simulink model "GunnerusDP_v1"  (R2017b)
settings: Solver=ode4  StartTime=0.0  StopTime=Tsim  FixedStep=ts  RelTol=1e-3  EnableMultiTasking=on
values from neighbouring files (symbols this model uses):
  ts = 0.01    [InitGunnerusDP.m]
undefined symbols (not defined in the file or in its folder): Control, Current, Hoerner, Par, Sim, TC_currentChange, vessel, vesselABC
libraries: marine_hydro x4, marine_gnc x3, simulink x3
(part 3 of 4)

== system GunnerusDP_v1/Environment and Vessel Dynamics/Wave definiton (from MCSim)/wave height and wave frequency/Hs and omega20/hs ==
  time : Inport
  Constant : Constant  Value=v1
  Constant2 : Constant  Value=v2
  If : If  IfExpression=u1 < t1  ElseIfExpressions=u1>=t1 & u1<t2
  If Action Subsystem1 : Subsystem  TreatAsAtomicUnit=on
  If Action Subsystem2 : Subsystem  TreatAsAtomicUnit=on
  If Action Subsystem3 : Subsystem  TreatAsAtomicUnit=on
  Merge : Merge  Inputs=3
  omega_peak : Outport
  wires:
  time/1 -> If Action Subsystem2/1(In1), If/1
  If/3 -> If Action Subsystem3/Action
  If/1 -> If Action Subsystem1/Action
  Constant/1 -> If Action Subsystem1/1(In1)
  Constant2/1 -> If Action Subsystem3/1(In1)
  If Action Subsystem3/1(Out1) -> Merge/3
  If Action Subsystem2/1(Out1) -> Merge/2
  If/2 -> If Action Subsystem2/Action
  If Action Subsystem1/1(Out1) -> Merge/1
  Merge/1 -> omega_peak/1

== system GunnerusDP_v1/Environment and Vessel Dynamics/Wave definiton (from MCSim)/wave height and wave frequency/Hs and omega20/omega_p ==
  time : Inport
  Constant : Constant  Value=v1
  Constant2 : Constant  Value=v2
  If : If  IfExpression=u1 < t1  ElseIfExpressions=u1>=t1 & u1<t2
  If Action Subsystem1 : Subsystem  TreatAsAtomicUnit=on
  If Action Subsystem2 : Subsystem  TreatAsAtomicUnit=on
  If Action Subsystem3 : Subsystem  TreatAsAtomicUnit=on
  Merge : Merge  Inputs=3
  omega_peak : Outport
  wires:
  Merge/1 -> omega_peak/1
  If Action Subsystem1/1(Out1) -> Merge/1
  If/2 -> If Action Subsystem2/Action
  If Action Subsystem2/1(Out1) -> Merge/2
  If Action Subsystem3/1(Out1) -> Merge/3
  Constant2/1 -> If Action Subsystem3/1(In1)
  Constant/1 -> If Action Subsystem1/1(In1)
  If/1 -> If Action Subsystem1/Action
  If/3 -> If Action Subsystem3/Action
  time/1 -> If/1, If Action Subsystem2/1(In1)

== system GunnerusDP_v1/Environment and Vessel Dynamics/Wave definiton (from MCSim)/wave height and wave frequency/Hs and omega21/hs ==
  time : Inport
  Constant : Constant  Value=v1
  Constant2 : Constant  Value=v2
  If : If  IfExpression=u1 < t1  ElseIfExpressions=u1>=t1 & u1<t2
  If Action Subsystem1 : Subsystem  TreatAsAtomicUnit=on
  If Action Subsystem2 : Subsystem  TreatAsAtomicUnit=on
  If Action Subsystem3 : Subsystem  TreatAsAtomicUnit=on
  Merge : Merge  Inputs=3
  omega_peak : Outport
  wires:
  Merge/1 -> omega_peak/1
  If Action Subsystem1/1(Out1) -> Merge/1
  If/2 -> If Action Subsystem2/Action
  If Action Subsystem2/1(Out1) -> Merge/2
  If Action Subsystem3/1(Out1) -> Merge/3
  Constant2/1 -> If Action Subsystem3/1(In1)
  Constant/1 -> If Action Subsystem1/1(In1)
  If/1 -> If Action Subsystem1/Action
  If/3 -> If Action Subsystem3/Action
  time/1 -> If/1, If Action Subsystem2/1(In1)

== system GunnerusDP_v1/Environment and Vessel Dynamics/Wave definiton (from MCSim)/wave height and wave frequency/Hs and omega21/omega_p ==
  time : Inport
  Constant : Constant  Value=v1
  Constant2 : Constant  Value=v2
  If : If  IfExpression=u1 < t1  ElseIfExpressions=u1>=t1 & u1<t2
  If Action Subsystem1 : Subsystem  TreatAsAtomicUnit=on
  If Action Subsystem2 : Subsystem  TreatAsAtomicUnit=on
  If Action Subsystem3 : Subsystem  TreatAsAtomicUnit=on
  Merge : Merge  Inputs=3
  omega_peak : Outport
  wires:
  time/1 -> If Action Subsystem2/1(In1), If/1
  If/3 -> If Action Subsystem3/Action
  If/1 -> If Action Subsystem1/Action
  Constant/1 -> If Action Subsystem1/1(In1)
  Constant2/1 -> If Action Subsystem3/1(In1)
  If Action Subsystem3/1(Out1) -> Merge/3
  If Action Subsystem2/1(Out1) -> Merge/2
  If/2 -> If Action Subsystem2/Action
  If Action Subsystem1/1(Out1) -> Merge/1
  Merge/1 -> omega_peak/1

== system GunnerusDP_v1/Environment and Vessel Dynamics/Wave definiton (from MCSim)/wave height and wave frequency/Hs and omega22/hs ==
  time : Inport
  Constant : Constant  Value=v1
  Constant2 : Constant  Value=v2
  If : If  IfExpression=u1 < t1  ElseIfExpressions=u1>=t1 & u1<t2
  If Action Subsystem1 : Subsystem  TreatAsAtomicUnit=on
  If Action Subsystem2 : Subsystem  TreatAsAtomicUnit=on
  If Action Subsystem3 : Subsystem  TreatAsAtomicUnit=on
  Merge : Merge  Inputs=3
  omega_peak : Outport
  wires:
  time/1 -> If Action Subsystem2/1(In1), If/1
  If/3 -> If Action Subsystem3/Action
  If/1 -> If Action Subsystem1/Action
  Constant/1 -> If Action Subsystem1/1(In1)
  Constant2/1 -> If Action Subsystem3/1(In1)
  If Action Subsystem3/1(Out1) -> Merge/3
  If Action Subsystem2/1(Out1) -> Merge/2
  If/2 -> If Action Subsystem2/Action
  If Action Subsystem1/1(Out1) -> Merge/1
  Merge/1 -> omega_peak/1

== system GunnerusDP_v1/Environment and Vessel Dynamics/Wave definiton (from MCSim)/wave height and wave frequency/Hs and omega22/omega_p ==
  time : Inport
  Constant : Constant  Value=v1
  Constant2 : Constant  Value=v2
  If : If  IfExpression=u1 < t1  ElseIfExpressions=u1>=t1 & u1<t2
  If Action Subsystem1 : Subsystem  TreatAsAtomicUnit=on
  If Action Subsystem2 : Subsystem  TreatAsAtomicUnit=on
  If Action Subsystem3 : Subsystem  TreatAsAtomicUnit=on
  Merge : Merge  Inputs=3
  omega_peak : Outport
  wires:
  Merge/1 -> omega_peak/1
  If Action Subsystem1/1(Out1) -> Merge/1
  If/2 -> If Action Subsystem2/Action
  If Action Subsystem2/1(Out1) -> Merge/2
  If Action Subsystem3/1(Out1) -> Merge/3
  Constant2/1 -> If Action Subsystem3/1(In1)
  Constant/1 -> If Action Subsystem1/1(In1)
  If/1 -> If Action Subsystem1/Action
  If/3 -> If Action Subsystem3/Action
  time/1 -> If/1, If Action Subsystem2/1(In1)

== system GunnerusDP_v1/Environment and Vessel Dynamics/Wave definiton (from MCSim)/wave height and wave frequency/Hs and omega23/hs ==
  time : Inport
  Constant : Constant  Value=v1
  Constant2 : Constant  Value=v2
  If : If  IfExpression=u1 < t1  ElseIfExpressions=u1>=t1 & u1<t2
  If Action Subsystem1 : Subsystem  TreatAsAtomicUnit=on
  If Action Subsystem2 : Subsystem  TreatAsAtomicUnit=on
  If Action Subsystem3 : Subsystem  TreatAsAtomicUnit=on
  Merge : Merge  Inputs=3
  omega_peak : Outport
  wires:
  Merge/1 -> omega_peak/1
  If Action Subsystem1/1(Out1) -> Merge/1
  If/2 -> If Action Subsystem2/Action
  If Action Subsystem2/1(Out1) -> Merge/2
  If Action Subsystem3/1(Out1) -> Merge/3
  Constant2/1 -> If Action Subsystem3/1(In1)
  Constant/1 -> If Action Subsystem1/1(In1)
  If/1 -> If Action Subsystem1/Action
  If/3 -> If Action Subsystem3/Action
  time/1 -> If/1, If Action Subsystem2/1(In1)

== system GunnerusDP_v1/Environment and Vessel Dynamics/Wave definiton (from MCSim)/wave height and wave frequency/Hs and omega23/omega_p ==
  time : Inport
  Constant : Constant  Value=v1
  Constant2 : Constant  Value=v2
  If : If  IfExpression=u1 < t1  ElseIfExpressions=u1>=t1 & u1<t2
  If Action Subsystem1 : Subsystem  TreatAsAtomicUnit=on
  If Action Subsystem2 : Subsystem  TreatAsAtomicUnit=on
  If Action Subsystem3 : Subsystem  TreatAsAtomicUnit=on
  Merge : Merge  Inputs=3
  omega_peak : Outport
  wires:
  time/1 -> If Action Subsystem2/1(In1), If/1
  If/3 -> If Action Subsystem3/Action
  If/1 -> If Action Subsystem1/Action
  Constant/1 -> If Action Subsystem1/1(In1)
  Constant2/1 -> If Action Subsystem3/1(In1)
  If Action Subsystem3/1(Out1) -> Merge/3
  If Action Subsystem2/1(Out1) -> Merge/2
  If/2 -> If Action Subsystem2/Action
  If Action Subsystem1/1(Out1) -> Merge/1
  Merge/1 -> omega_peak/1

== system GunnerusDP_v1/Environment and Vessel Dynamics/Wave definiton (from MCSim)/wave height and wave frequency/Hs and omega24/hs ==
  time : Inport
  Constant : Constant  Value=v1
  Constant2 : Constant  Value=v2
  If : If  IfExpression=u1 < t1  ElseIfExpressions=u1>=t1 & u1<t2
  If Action Subsystem1 : Subsystem  TreatAsAtomicUnit=on
  If Action Subsystem2 : Subsystem  TreatAsAtomicUnit=on
  If Action Subsystem3 : Subsystem  TreatAsAtomicUnit=on
  Merge : Merge  Inputs=3
  omega_peak : Outport
  wires:
  time/1 -> If Action Subsystem2/1(In1), If/1
  If/3 -> If Action Subsystem3/Action
  If/1 -> If Action Subsystem1/Action
  Constant/1 -> If Action Subsystem1/1(In1)
  Constant2/1 -> If Action Subsystem3/1(In1)
  If Action Subsystem3/1(Out1) -> Merge/3
  If Action Subsystem2/1(Out1) -> Merge/2
  If/2 -> If Action Subsystem2/Action
  If Action Subsystem1/1(Out1) -> Merge/1
  Merge/1 -> omega_peak/1

== system GunnerusDP_v1/Environment and Vessel Dynamics/Wave definiton (from MCSim)/wave height and wave frequency/Hs and omega24/omega_p ==
  time : Inport
  Constant : Constant  Value=v1
  Constant2 : Constant  Value=v2
  If : If  IfExpression=u1 < t1  ElseIfExpressions=u1>=t1 & u1<t2
  If Action Subsystem1 : Subsystem  TreatAsAtomicUnit=on
  If Action Subsystem2 : Subsystem  TreatAsAtomicUnit=on
  If Action Subsystem3 : Subsystem  TreatAsAtomicUnit=on
  Merge : Merge  Inputs=3
  omega_peak : Outport
  wires:
  Merge/1 -> omega_peak/1
  If Action Subsystem1/1(Out1) -> Merge/1
  If/2 -> If Action Subsystem2/Action
  If Action Subsystem2/1(Out1) -> Merge/2
  If Action Subsystem3/1(Out1) -> Merge/3
  Constant2/1 -> If Action Subsystem3/1(In1)
  Constant/1 -> If Action Subsystem1/1(In1)
  If/1 -> If Action Subsystem1/Action
  If/3 -> If Action Subsystem3/Action
  time/1 -> If/1, If Action Subsystem2/1(In1)

== system GunnerusDP_v1/Environment and Vessel Dynamics/Wave definiton (from MCSim)/wave height and wave frequency/Hs and omega3/hs ==
  time : Inport
  Constant : Constant  Value=v1
  Constant2 : Constant  Value=v2
  If : If  IfExpression=u1 < t1  ElseIfExpressions=u1>=t1 & u1<t2
  If Action Subsystem1 : Subsystem  TreatAsAtomicUnit=on
  If Action Subsystem2 : Subsystem  TreatAsAtomicUnit=on
  If Action Subsystem3 : Subsystem  TreatAsAtomicUnit=on
  Merge : Merge  Inputs=3
  omega_peak : Outport
  wires:
  time/1 -> If Action Subsystem2/1(In1), If/1
  If/3 -> If Action Subsystem3/Action
  If/1 -> If Action Subsystem1/Action
  Constant/1 -> If Action Subsystem1/1(In1)
  Constant2/1 -> If Action Subsystem3/1(In1)
  If Action Subsystem3/1(Out1) -> Merge/3
  If Action Subsystem2/1(Out1) -> Merge/2
  If/2 -> If Action Subsystem2/Action
  If Action Subsystem1/1(Out1) -> Merge/1
  Merge/1 -> omega_peak/1

== system GunnerusDP_v1/Environment and Vessel Dynamics/Wave definiton (from MCSim)/wave height and wave frequency/Hs and omega3/omega_p ==
  time : Inport
  Constant : Constant  Value=v1
  Constant2 : Constant  Value=v2
  If : If  IfExpression=u1 < t1  ElseIfExpressions=u1>=t1 & u1<t2
  If Action Subsystem1 : Subsystem  TreatAsAtomicUnit=on
  If Action Subsystem2 : Subsystem  TreatAsAtomicUnit=on
  If Action Subsystem3 : Subsystem  TreatAsAtomicUnit=on
  Merge : Merge  Inputs=3
  omega_peak : Outport
  wires:
  Merge/1 -> omega_peak/1
  If Action Subsystem1/1(Out1) -> Merge/1
  If/2 -> If Action Subsystem2/Action
  If Action Subsystem2/1(Out1) -> Merge/2
  If Action Subsystem3/1(Out1) -> Merge/3
  Constant2/1 -> If Action Subsystem3/1(In1)
  Constant/1 -> If Action Subsystem1/1(In1)
  If/1 -> If Action Subsystem1/Action
  If/3 -> If Action Subsystem3/Action
  time/1 -> If/1, If Action Subsystem2/1(In1)

== system GunnerusDP_v1/Environment and Vessel Dynamics/Wave definiton (from MCSim)/wave height and wave frequency/Hs and omega4/hs ==
  time : Inport
  Constant : Constant  Value=v1
  Constant2 : Constant  Value=v2
  If : If  IfExpression=u1 < t1  ElseIfExpressions=u1>=t1 & u1<t2
  If Action Subsystem1 : Subsystem  TreatAsAtomicUnit=on
  If Action Subsystem2 : Subsystem  TreatAsAtomicUnit=on
  If Action Subsystem3 : Subsystem  TreatAsAtomicUnit=on
  Merge : Merge  Inputs=3
  omega_peak : Outport
  wires:
  Merge/1 -> omega_peak/1
  If Action Subsystem1/1(Out1) -> Merge/1
  If/2 -> If Action Subsystem2/Action
  If Action Subsystem2/1(Out1) -> Merge/2
  If Action Subsystem3/1(Out1) -> Merge/3
  Constant2/1 -> If Action Subsystem3/1(In1)
  Constant/1 -> If Action Subsystem1/1(In1)
  If/1 -> If Action Subsystem1/Action
  If/3 -> If Action Subsystem3/Action
  time/1 -> If/1, If Action Subsystem2/1(In1)

== system GunnerusDP_v1/Environment and Vessel Dynamics/Wave definiton (from MCSim)/wave height and wave frequency/Hs and omega4/omega_p ==
  time : Inport
  Constant : Constant  Value=v1
  Constant2 : Constant  Value=v2
  If : If  IfExpression=u1 < t1  ElseIfExpressions=u1>=t1 & u1<t2
  If Action Subsystem1 : Subsystem  TreatAsAtomicUnit=on
  If Action Subsystem2 : Subsystem  TreatAsAtomicUnit=on
  If Action Subsystem3 : Subsystem  TreatAsAtomicUnit=on
  Merge : Merge  Inputs=3
  omega_peak : Outport
  wires:
  time/1 -> If Action Subsystem2/1(In1), If/1
  If/3 -> If Action Subsystem3/Action
  If/1 -> If Action Subsystem1/Action
  Constant/1 -> If Action Subsystem1/1(In1)
  Constant2/1 -> If Action Subsystem3/1(In1)
  If Action Subsystem3/1(Out1) -> Merge/3
  If Action Subsystem2/1(Out1) -> Merge/2
  If/2 -> If Action Subsystem2/Action
  If Action Subsystem1/1(Out1) -> Merge/1
  Merge/1 -> omega_peak/1

== system GunnerusDP_v1/Environment and Vessel Dynamics/Wave definiton (from MCSim)/wave height and wave frequency/Hs and omega5/hs ==
  time : Inport
  Constant : Constant  Value=v1
  Constant2 : Constant  Value=v2
  If : If  IfExpression=u1 < t1  ElseIfExpressions=u1>=t1 & u1<t2
  If Action Subsystem1 : Subsystem  TreatAsAtomicUnit=on
  If Action Subsystem2 : Subsystem  TreatAsAtomicUnit=on
  If Action Subsystem3 : Subsystem  TreatAsAtomicUnit=on
  Merge : Merge  Inputs=3
  omega_peak : Outport
  wires:
  time/1 -> If Action Subsystem2/1(In1), If/1
  If/3 -> If Action Subsystem3/Action
  If/1 -> If Action Subsystem1/Action
  Constant/1 -> If Action Subsystem1/1(In1)
  Constant2/1 -> If Action Subsystem3/1(In1)
  If Action Subsystem3/1(Out1) -> Merge/3
  If Action Subsystem2/1(Out1) -> Merge/2
  If/2 -> If Action Subsystem2/Action
  If Action Subsystem1/1(Out1) -> Merge/1
  Merge/1 -> omega_peak/1

== system GunnerusDP_v1/Environment and Vessel Dynamics/Wave definiton (from MCSim)/wave height and wave frequency/Hs and omega5/omega_p ==
  time : Inport
  Constant : Constant  Value=v1
  Constant2 : Constant  Value=v2
  If : If  IfExpression=u1 < t1  ElseIfExpressions=u1>=t1 & u1<t2
  If Action Subsystem1 : Subsystem  TreatAsAtomicUnit=on
  If Action Subsystem2 : Subsystem  TreatAsAtomicUnit=on
  If Action Subsystem3 : Subsystem  TreatAsAtomicUnit=on
  Merge : Merge  Inputs=3
  omega_peak : Outport
  wires:
  Merge/1 -> omega_peak/1
  If Action Subsystem1/1(Out1) -> Merge/1
  If/2 -> If Action Subsystem2/Action
  If Action Subsystem2/1(Out1) -> Merge/2
  If Action Subsystem3/1(Out1) -> Merge/3
  Constant2/1 -> If Action Subsystem3/1(In1)
  Constant/1 -> If Action Subsystem1/1(In1)
  If/1 -> If Action Subsystem1/Action
  If/3 -> If Action Subsystem3/Action
  time/1 -> If/1, If Action Subsystem2/1(In1)

== system GunnerusDP_v1/Environment and Vessel Dynamics/Wave definiton (from MCSim)/wave height and wave frequency/Hs and omega6/hs ==
  time : Inport
  Constant : Constant  Value=v1
  Constant2 : Constant  Value=v2
  If : If  IfExpression=u1 < t1  ElseIfExpressions=u1>=t1 & u1<t2
  If Action Subsystem1 : Subsystem  TreatAsAtomicUnit=on
  If Action Subsystem2 : Subsystem  TreatAsAtomicUnit=on
  If Action Subsystem3 : Subsystem  TreatAsAtomicUnit=on
  Merge : Merge  Inputs=3
  omega_peak : Outport
  wires:
  Merge/1 -> omega_peak/1
  If Action Subsystem1/1(Out1) -> Merge/1
  If/2 -> If Action Subsystem2/Action
  If Action Subsystem2/1(Out1) -> Merge/2
  If Action Subsystem3/1(Out1) -> Merge/3
  Constant2/1 -> If Action Subsystem3/1(In1)
  Constant/1 -> If Action Subsystem1/1(In1)
  If/1 -> If Action Subsystem1/Action
  If/3 -> If Action Subsystem3/Action
  time/1 -> If/1, If Action Subsystem2/1(In1)

== system GunnerusDP_v1/Environment and Vessel Dynamics/Wave definiton (from MCSim)/wave height and wave frequency/Hs and omega6/omega_p ==
  time : Inport
  Constant : Constant  Value=v1
  Constant2 : Constant  Value=v2
  If : If  IfExpression=u1 < t1  ElseIfExpressions=u1>=t1 & u1<t2
  If Action Subsystem1 : Subsystem  TreatAsAtomicUnit=on
  If Action Subsystem2 : Subsystem  TreatAsAtomicUnit=on
  If Action Subsystem3 : Subsystem  TreatAsAtomicUnit=on
  Merge : Merge  Inputs=3
  omega_peak : Outport
  wires:
  time/1 -> If Action Subsystem2/1(In1), If/1
  If/3 -> If Action Subsystem3/Action
  If/1 -> If Action Subsystem1/Action
  Constant/1 -> If Action Subsystem1/1(In1)
  Constant2/1 -> If Action Subsystem3/1(In1)
  If Action Subsystem3/1(Out1) -> Merge/3
  If Action Subsystem2/1(Out1) -> Merge/2
  If/2 -> If Action Subsystem2/Action
  If Action Subsystem1/1(Out1) -> Merge/1
  Merge/1 -> omega_peak/1

== system GunnerusDP_v1/Environment and Vessel Dynamics/Wave definiton (from MCSim)/wave height and wave frequency/Hs and omega7/hs ==
  time : Inport
  Constant : Constant  Value=v1
  Constant2 : Constant  Value=v2
  If : If  IfExpression=u1 < t1  ElseIfExpressions=u1>=t1 & u1<t2
  If Action Subsystem1 : Subsystem  TreatAsAtomicUnit=on
  If Action Subsystem2 : Subsystem  TreatAsAtomicUnit=on
  If Action Subsystem3 : Subsystem  TreatAsAtomicUnit=on
  Merge : Merge  Inputs=3
  omega_peak : Outport
  wires:
  time/1 -> If Action Subsystem2/1(In1), If/1
  If/3 -> If Action Subsystem3/Action
  If/1 -> If Action Subsystem1/Action
  Constant/1 -> If Action Subsystem1/1(In1)
  Constant2/1 -> If Action Subsystem3/1(In1)
  If Action Subsystem3/1(Out1) -> Merge/3
  If Action Subsystem2/1(Out1) -> Merge/2
  If/2 -> If Action Subsystem2/Action
  If Action Subsystem1/1(Out1) -> Merge/1
  Merge/1 -> omega_peak/1

== system GunnerusDP_v1/Environment and Vessel Dynamics/Wave definiton (from MCSim)/wave height and wave frequency/Hs and omega7/omega_p ==
  time : Inport
  Constant : Constant  Value=v1
  Constant2 : Constant  Value=v2
  If : If  IfExpression=u1 < t1  ElseIfExpressions=u1>=t1 & u1<t2
  If Action Subsystem1 : Subsystem  TreatAsAtomicUnit=on
  If Action Subsystem2 : Subsystem  TreatAsAtomicUnit=on
  If Action Subsystem3 : Subsystem  TreatAsAtomicUnit=on
  Merge : Merge  Inputs=3
  omega_peak : Outport
  wires:
  Merge/1 -> omega_peak/1
  If Action Subsystem1/1(Out1) -> Merge/1
  If/2 -> If Action Subsystem2/Action
  If Action Subsystem2/1(Out1) -> Merge/2
  If Action Subsystem3/1(Out1) -> Merge/3
  Constant2/1 -> If Action Subsystem3/1(In1)
  Constant/1 -> If Action Subsystem1/1(In1)
  If/1 -> If Action Subsystem1/Action
  If/3 -> If Action Subsystem3/Action
  time/1 -> If/1, If Action Subsystem2/1(In1)

== system GunnerusDP_v1/Environment and Vessel Dynamics/Wave definiton (from MCSim)/wave height and wave frequency/Hs and omega8/hs ==
  time : Inport
  Constant : Constant  Value=v1
  Constant2 : Constant  Value=v2
  If : If  IfExpression=u1 < t1  ElseIfExpressions=u1>=t1 & u1<t2
  If Action Subsystem1 : Subsystem  TreatAsAtomicUnit=on
  If Action Subsystem2 : Subsystem  TreatAsAtomicUnit=on
  If Action Subsystem3 : Subsystem  TreatAsAtomicUnit=on
  Merge : Merge  Inputs=3
  omega_peak : Outport
  wires:
  Merge/1 -> omega_peak/1
  If Action Subsystem1/1(Out1) -> Merge/1
  If/2 -> If Action Subsystem2/Action
  If Action Subsystem2/1(Out1) -> Merge/2
  If Action Subsystem3/1(Out1) -> Merge/3
  Constant2/1 -> If Action Subsystem3/1(In1)
  Constant/1 -> If Action Subsystem1/1(In1)
  If/1 -> If Action Subsystem1/Action
  If/3 -> If Action Subsystem3/Action
  time/1 -> If/1, If Action Subsystem2/1(In1)

== system GunnerusDP_v1/Environment and Vessel Dynamics/Wave definiton (from MCSim)/wave height and wave frequency/Hs and omega8/omega_p ==
  time : Inport
  Constant : Constant  Value=v1
  Constant2 : Constant  Value=v2
  If : If  IfExpression=u1 < t1  ElseIfExpressions=u1>=t1 & u1<t2
  If Action Subsystem1 : Subsystem  TreatAsAtomicUnit=on
  If Action Subsystem2 : Subsystem  TreatAsAtomicUnit=on
  If Action Subsystem3 : Subsystem  TreatAsAtomicUnit=on
  Merge : Merge  Inputs=3
  omega_peak : Outport
  wires:
  time/1 -> If Action Subsystem2/1(In1), If/1
  If/3 -> If Action Subsystem3/Action
  If/1 -> If Action Subsystem1/Action
  Constant/1 -> If Action Subsystem1/1(In1)
  Constant2/1 -> If Action Subsystem3/1(In1)
  If Action Subsystem3/1(Out1) -> Merge/3
  If Action Subsystem2/1(Out1) -> Merge/2
  If/2 -> If Action Subsystem2/Action
  If Action Subsystem1/1(Out1) -> Merge/1
  Merge/1 -> omega_peak/1

== system GunnerusDP_v1/Environment and Vessel Dynamics/Wave definiton (from MCSim)/wave height and wave frequency/Hs and omega9/hs ==
  time : Inport
  Constant : Constant  Value=v1
  Constant2 : Constant  Value=v2
  If : If  IfExpression=u1 < t1  ElseIfExpressions=u1>=t1 & u1<t2
  If Action Subsystem1 : Subsystem  TreatAsAtomicUnit=on
  If Action Subsystem2 : Subsystem  TreatAsAtomicUnit=on
  If Action Subsystem3 : Subsystem  TreatAsAtomicUnit=on
  Merge : Merge  Inputs=3
  omega_peak : Outport
  wires:
  time/1 -> If Action Subsystem2/1(In1), If/1
  If/3 -> If Action Subsystem3/Action
  If/1 -> If Action Subsystem1/Action
  Constant/1 -> If Action Subsystem1/1(In1)
  Constant2/1 -> If Action Subsystem3/1(In1)
  If Action Subsystem3/1(Out1) -> Merge/3
  If Action Subsystem2/1(Out1) -> Merge/2
  If/2 -> If Action Subsystem2/Action
  If Action Subsystem1/1(Out1) -> Merge/1
  Merge/1 -> omega_peak/1

== system GunnerusDP_v1/Environment and Vessel Dynamics/Wave definiton (from MCSim)/wave height and wave frequency/Hs and omega9/omega_p ==
  time : Inport
  Constant : Constant  Value=v1
  Constant2 : Constant  Value=v2
  If : If  IfExpression=u1 < t1  ElseIfExpressions=u1>=t1 & u1<t2
  If Action Subsystem1 : Subsystem  TreatAsAtomicUnit=on
  If Action Subsystem2 : Subsystem  TreatAsAtomicUnit=on
  If Action Subsystem3 : Subsystem  TreatAsAtomicUnit=on
  Merge : Merge  Inputs=3
  omega_peak : Outport
  wires:
  Merge/1 -> omega_peak/1
  If Action Subsystem1/1(Out1) -> Merge/1
  If/2 -> If Action Subsystem2/Action
  If Action Subsystem2/1(Out1) -> Merge/2
  If Action Subsystem3/1(Out1) -> Merge/3
  Constant2/1 -> If Action Subsystem3/1(In1)
  Constant/1 -> If Action Subsystem1/1(In1)
  If/1 -> If Action Subsystem1/Action
  If/3 -> If Action Subsystem3/Action
  time/1 -> If/1, If Action Subsystem2/1(In1)

== system GunnerusDP_v1/Environment and Vessel Dynamics/Wave definiton (from MCSim)/wave height and wave frequency/Hs and omega1/hs/If Action Subsystem1 ==
  In1 : Inport
  Action Port : ActionPort  ActionType=then
  Out1 : Outport
  wires:
  In1/1 -> Out1/1

== system GunnerusDP_v1/Environment and Vessel Dynamics/Wave definiton (from MCSim)/wave height and wave frequency/Hs and omega1/hs/If Action Subsystem2 ==
  In1 : Inport
  Action Port : ActionPort  ActionType=elseif
  Fcn : Fcn  Expr=v1-(v1-v2)/(t2-t1)*(u[1]-t1)
  Out1 : Outport
  wires:
  In1/1 -> Fcn/1
  Fcn/1 -> Out1/1

== system GunnerusDP_v1/Environment and Vessel Dynamics/Wave definiton (from MCSim)/wave height and wave frequency/Hs and omega1/hs/If Action Subsystem3 ==
  In1 : Inport
  Action Port : ActionPort  ActionType=else
  Out1 : Outport
  wires:
  In1/1 -> Out1/1

== system GunnerusDP_v1/Environment and Vessel Dynamics/Wave definiton (from MCSim)/wave height and wave frequency/Hs and omega1/omega_p/If Action Subsystem1 ==
  In1 : Inport
  Action Port : ActionPort  ActionType=then
  Out1 : Outport
  wires:
  In1/1 -> Out1/1

== system GunnerusDP_v1/Environment and Vessel Dynamics/Wave definiton (from MCSim)/wave height and wave frequency/Hs and omega1/omega_p/If Action Subsystem2 ==
  In1 : Inport
  Action Port : ActionPort  ActionType=elseif
  Fcn : Fcn  Expr=v1-(v1-v2)/(t2-t1)*(u[1]-t1)
  Out1 : Outport
  wires:
  Fcn/1 -> Out1/1
  In1/1 -> Fcn/1

== system GunnerusDP_v1/Environment and Vessel Dynamics/Wave definiton (from MCSim)/wave height and wave frequency/Hs and omega1/omega_p/If Action Subsystem3 ==
  In1 : Inport
  Action Port : ActionPort  ActionType=else
  Out1 : Outport
  wires:
  In1/1 -> Out1/1

== system GunnerusDP_v1/Environment and Vessel Dynamics/Wave definiton (from MCSim)/wave height and wave frequency/Hs and omega10/hs/If Action Subsystem1 ==
  In1 : Inport
  Action Port : ActionPort  ActionType=then
  Out1 : Outport
  wires:
  In1/1 -> Out1/1

== system GunnerusDP_v1/Environment and Vessel Dynamics/Wave definiton (from MCSim)/wave height and wave frequency/Hs and omega10/hs/If Action Subsystem2 ==
  In1 : Inport
  Action Port : ActionPort  ActionType=elseif
  Fcn : Fcn  Expr=v1-(v1-v2)/(t2-t1)*(u[1]-t1)
  Out1 : Outport
  wires:
  Fcn/1 -> Out1/1
  In1/1 -> Fcn/1

== system GunnerusDP_v1/Environment and Vessel Dynamics/Wave definiton (from MCSim)/wave height and wave frequency/Hs and omega10/hs/If Action Subsystem3 ==
  In1 : Inport
  Action Port : ActionPort  ActionType=else
  Out1 : Outport
  wires:
  In1/1 -> Out1/1

== system GunnerusDP_v1/Environment and Vessel Dynamics/Wave definiton (from MCSim)/wave height and wave frequency/Hs and omega10/omega_p/If Action Subsystem1 ==
  In1 : Inport
  Action Port : ActionPort  ActionType=then
  Out1 : Outport
  wires:
  In1/1 -> Out1/1

== system GunnerusDP_v1/Environment and Vessel Dynamics/Wave definiton (from MCSim)/wave height and wave frequency/Hs and omega10/omega_p/If Action Subsystem2 ==
  In1 : Inport
  Action Port : ActionPort  ActionType=elseif
  Fcn : Fcn  Expr=v1-(v1-v2)/(t2-t1)*(u[1]-t1)
  Out1 : Outport
  wires:
  In1/1 -> Fcn/1
  Fcn/1 -> Out1/1

== system GunnerusDP_v1/Environment and Vessel Dynamics/Wave definiton (from MCSim)/wave height and wave frequency/Hs and omega10/omega_p/If Action Subsystem3 ==
  In1 : Inport
  Action Port : ActionPort  ActionType=else
  Out1 : Outport
  wires:
  In1/1 -> Out1/1

== system GunnerusDP_v1/Environment and Vessel Dynamics/Wave definiton (from MCSim)/wave height and wave frequency/Hs and omega11/hs/If Action Subsystem1 ==
  In1 : Inport
  Action Port : ActionPort  ActionType=then
  Out1 : Outport
  wires:
  In1/1 -> Out1/1

== system GunnerusDP_v1/Environment and Vessel Dynamics/Wave definiton (from MCSim)/wave height and wave frequency/Hs and omega11/hs/If Action Subsystem2 ==
  In1 : Inport
  Action Port : ActionPort  ActionType=elseif
  Fcn : Fcn  Expr=v1-(v1-v2)/(t2-t1)*(u[1]-t1)
  Out1 : Outport
  wires:
  In1/1 -> Fcn/1
  Fcn/1 -> Out1/1

== system GunnerusDP_v1/Environment and Vessel Dynamics/Wave definiton (from MCSim)/wave height and wave frequency/Hs and omega11/hs/If Action Subsystem3 ==
  In1 : Inport
  Action Port : ActionPort  ActionType=else
  Out1 : Outport
  wires:
  In1/1 -> Out1/1

== system GunnerusDP_v1/Environment and Vessel Dynamics/Wave definiton (from MCSim)/wave height and wave frequency/Hs and omega11/omega_p/If Action Subsystem1 ==
  In1 : Inport
  Action Port : ActionPort  ActionType=then
  Out1 : Outport
  wires:
  In1/1 -> Out1/1

== system GunnerusDP_v1/Environment and Vessel Dynamics/Wave definiton (from MCSim)/wave height and wave frequency/Hs and omega11/omega_p/If Action Subsystem2 ==
  In1 : Inport
  Action Port : ActionPort  ActionType=elseif
  Fcn : Fcn  Expr=v1-(v1-v2)/(t2-t1)*(u[1]-t1)
  Out1 : Outport
  wires:
  Fcn/1 -> Out1/1
  In1/1 -> Fcn/1

== system GunnerusDP_v1/Environment and Vessel Dynamics/Wave definiton (from MCSim)/wave height and wave frequency/Hs and omega11/omega_p/If Action Subsystem3 ==
  In1 : Inport
  Action Port : ActionPort  ActionType=else
  Out1 : Outport
  wires:
  In1/1 -> Out1/1

== system GunnerusDP_v1/Environment and Vessel Dynamics/Wave definiton (from MCSim)/wave height and wave frequency/Hs and omega12/hs/If Action Subsystem1 ==
  In1 : Inport
  Action Port : ActionPort  ActionType=then
  Out1 : Outport
  wires:
  In1/1 -> Out1/1

== system GunnerusDP_v1/Environment and Vessel Dynamics/Wave definiton (from MCSim)/wave height and wave frequency/Hs and omega12/hs/If Action Subsystem2 ==
  In1 : Inport
  Action Port : ActionPort  ActionType=elseif
  Fcn : Fcn  Expr=v1-(v1-v2)/(t2-t1)*(u[1]-t1)
  Out1 : Outport
  wires:
  Fcn/1 -> Out1/1
  In1/1 -> Fcn/1

== system GunnerusDP_v1/Environment and Vessel Dynamics/Wave definiton (from MCSim)/wave height and wave frequency/Hs and omega12/hs/If Action Subsystem3 ==
  In1 : Inport
  Action Port : ActionPort  ActionType=else
  Out1 : Outport
  wires:
  In1/1 -> Out1/1

== system GunnerusDP_v1/Environment and Vessel Dynamics/Wave definiton (from MCSim)/wave height and wave frequency/Hs and omega12/omega_p/If Action Subsystem1 ==
  In1 : Inport
  Action Port : ActionPort  ActionType=then
  Out1 : Outport
  wires:
  In1/1 -> Out1/1

== system GunnerusDP_v1/Environment and Vessel Dynamics/Wave definiton (from MCSim)/wave height and wave frequency/Hs and omega12/omega_p/If Action Subsystem2 ==
  In1 : Inport
  Action Port : ActionPort  ActionType=elseif
  Fcn : Fcn  Expr=v1-(v1-v2)/(t2-t1)*(u[1]-t1)
  Out1 : Outport
  wires:
  In1/1 -> Fcn/1
  Fcn/1 -> Out1/1

== system GunnerusDP_v1/Environment and Vessel Dynamics/Wave definiton (from MCSim)/wave height and wave frequency/Hs and omega12/omega_p/If Action Subsystem3 ==
  In1 : Inport
  Action Port : ActionPort  ActionType=else
  Out1 : Outport
  wires:
  In1/1 -> Out1/1

== system GunnerusDP_v1/Environment and Vessel Dynamics/Wave definiton (from MCSim)/wave height and wave frequency/Hs and omega13/hs/If Action Subsystem1 ==
  In1 : Inport
  Action Port : ActionPort  ActionType=then
  Out1 : Outport
  wires:
  In1/1 -> Out1/1

== system GunnerusDP_v1/Environment and Vessel Dynamics/Wave definiton (from MCSim)/wave height and wave frequency/Hs and omega13/hs/If Action Subsystem2 ==
  In1 : Inport
  Action Port : ActionPort  ActionType=elseif
  Fcn : Fcn  Expr=v1-(v1-v2)/(t2-t1)*(u[1]-t1)
  Out1 : Outport
  wires:
  In1/1 -> Fcn/1
  Fcn/1 -> Out1/1

== system GunnerusDP_v1/Environment and Vessel Dynamics/Wave definiton (from MCSim)/wave height and wave frequency/Hs and omega13/hs/If Action Subsystem3 ==
  In1 : Inport
  Action Port : ActionPort  ActionType=else
  Out1 : Outport
  wires:
  In1/1 -> Out1/1

== system GunnerusDP_v1/Environment and Vessel Dynamics/Wave definiton (from MCSim)/wave height and wave frequency/Hs and omega13/omega_p/If Action Subsystem1 ==
  In1 : Inport
  Action Port : ActionPort  ActionType=then
  Out1 : Outport
  wires:
  In1/1 -> Out1/1

== system GunnerusDP_v1/Environment and Vessel Dynamics/Wave definiton (from MCSim)/wave height and wave frequency/Hs and omega13/omega_p/If Action Subsystem2 ==
  In1 : Inport
  Action Port : ActionPort  ActionType=elseif
  Fcn : Fcn  Expr=v1-(v1-v2)/(t2-t1)*(u[1]-t1)
  Out1 : Outport
  wires:
  Fcn/1 -> Out1/1
  In1/1 -> Fcn/1

== system GunnerusDP_v1/Environment and Vessel Dynamics/Wave definiton (from MCSim)/wave height and wave frequency/Hs and omega13/omega_p/If Action Subsystem3 ==
  In1 : Inport
  Action Port : ActionPort  ActionType=else
  Out1 : Outport
  wires:
  In1/1 -> Out1/1

== system GunnerusDP_v1/Environment and Vessel Dynamics/Wave definiton (from MCSim)/wave height and wave frequency/Hs and omega14/hs/If Action Subsystem1 ==
  In1 : Inport
  Action Port : ActionPort  ActionType=then
  Out1 : Outport
  wires:
  In1/1 -> Out1/1

== system GunnerusDP_v1/Environment and Vessel Dynamics/Wave definiton (from MCSim)/wave height and wave frequency/Hs and omega14/hs/If Action Subsystem2 ==
  In1 : Inport
  Action Port : ActionPort  ActionType=elseif
  Fcn : Fcn  Expr=v1-(v1-v2)/(t2-t1)*(u[1]-t1)
  Out1 : Outport
  wires:
  Fcn/1 -> Out1/1
  In1/1 -> Fcn/1

== system GunnerusDP_v1/Environment and Vessel Dynamics/Wave definiton (from MCSim)/wave height and wave frequency/Hs and omega14/hs/If Action Subsystem3 ==
  In1 : Inport
  Action Port : ActionPort  ActionType=else
  Out1 : Outport
  wires:
  In1/1 -> Out1/1

== system GunnerusDP_v1/Environment and Vessel Dynamics/Wave definiton (from MCSim)/wave height and wave frequency/Hs and omega14/omega_p/If Action Subsystem1 ==
  In1 : Inport
  Action Port : ActionPort  ActionType=then
  Out1 : Outport
  wires:
  In1/1 -> Out1/1

== system GunnerusDP_v1/Environment and Vessel Dynamics/Wave definiton (from MCSim)/wave height and wave frequency/Hs and omega14/omega_p/If Action Subsystem2 ==
  In1 : Inport
  Action Port : ActionPort  ActionType=elseif
  Fcn : Fcn  Expr=v1-(v1-v2)/(t2-t1)*(u[1]-t1)
  Out1 : Outport
  wires:
  In1/1 -> Fcn/1
  Fcn/1 -> Out1/1

== system GunnerusDP_v1/Environment and Vessel Dynamics/Wave definiton (from MCSim)/wave height and wave frequency/Hs and omega14/omega_p/If Action Subsystem3 ==
  In1 : Inport
  Action Port : ActionPort  ActionType=else
  Out1 : Outport
  wires:
  In1/1 -> Out1/1

== system GunnerusDP_v1/Environment and Vessel Dynamics/Wave definiton (from MCSim)/wave height and wave frequency/Hs and omega15/hs/If Action Subsystem1 ==
  In1 : Inport
  Action Port : ActionPort  ActionType=then
  Out1 : Outport
  wires:
  In1/1 -> Out1/1

== system GunnerusDP_v1/Environment and Vessel Dynamics/Wave definiton (from MCSim)/wave height and wave frequency/Hs and omega15/hs/If Action Subsystem2 ==
  In1 : Inport
  Action Port : ActionPort  ActionType=elseif
  Fcn : Fcn  Expr=v1-(v1-v2)/(t2-t1)*(u[1]-t1)
  Out1 : Outport
  wires:
  In1/1 -> Fcn/1
  Fcn/1 -> Out1/1

== system GunnerusDP_v1/Environment and Vessel Dynamics/Wave definiton (from MCSim)/wave height and wave frequency/Hs and omega15/hs/If Action Subsystem3 ==
  In1 : Inport
  Action Port : ActionPort  ActionType=else
  Out1 : Outport
  wires:
  In1/1 -> Out1/1

== system GunnerusDP_v1/Environment and Vessel Dynamics/Wave definiton (from MCSim)/wave height and wave frequency/Hs and omega15/omega_p/If Action Subsystem1 ==
  In1 : Inport
  Action Port : ActionPort  ActionType=then
  Out1 : Outport
  wires:
  In1/1 -> Out1/1

== system GunnerusDP_v1/Environment and Vessel Dynamics/Wave definiton (from MCSim)/wave height and wave frequency/Hs and omega15/omega_p/If Action Subsystem2 ==
  In1 : Inport
  Action Port : ActionPort  ActionType=elseif
  Fcn : Fcn  Expr=v1-(v1-v2)/(t2-t1)*(u[1]-t1)
  Out1 : Outport
  wires:
  Fcn/1 -> Out1/1
  In1/1 -> Fcn/1

== system GunnerusDP_v1/Environment and Vessel Dynamics/Wave definiton (from MCSim)/wave height and wave frequency/Hs and omega15/omega_p/If Action Subsystem3 ==
  In1 : Inport
  Action Port : ActionPort  ActionType=else
  Out1 : Outport
  wires:
  In1/1 -> Out1/1

== system GunnerusDP_v1/Environment and Vessel Dynamics/Wave definiton (from MCSim)/wave height and wave frequency/Hs and omega16/hs/If Action Subsystem1 ==
  In1 : Inport
  Action Port : ActionPort  ActionType=then
  Out1 : Outport
  wires:
  In1/1 -> Out1/1

== system GunnerusDP_v1/Environment and Vessel Dynamics/Wave definiton (from MCSim)/wave height and wave frequency/Hs and omega16/hs/If Action Subsystem2 ==
  In1 : Inport
  Action Port : ActionPort  ActionType=elseif
  Fcn : Fcn  Expr=v1-(v1-v2)/(t2-t1)*(u[1]-t1)
  Out1 : Outport
  wires:
  In1/1 -> Fcn/1
  Fcn/1 -> Out1/1

== system GunnerusDP_v1/Environment and Vessel Dynamics/Wave definiton (from MCSim)/wave height and wave frequency/Hs and omega16/hs/If Action Subsystem3 ==
  In1 : Inport
  Action Port : ActionPort  ActionType=else
  Out1 : Outport
  wires:
  In1/1 -> Out1/1

== system GunnerusDP_v1/Environment and Vessel Dynamics/Wave definiton (from MCSim)/wave height and wave frequency/Hs and omega16/omega_p/If Action Subsystem1 ==
  In1 : Inport
  Action Port : ActionPort  ActionType=then
  Out1 : Outport
  wires:
  In1/1 -> Out1/1

== system GunnerusDP_v1/Environment and Vessel Dynamics/Wave definiton (from MCSim)/wave height and wave frequency/Hs and omega16/omega_p/If Action Subsystem2 ==
  In1 : Inport
  Action Port : ActionPort  ActionType=elseif
  Fcn : Fcn  Expr=v1-(v1-v2)/(t2-t1)*(u[1]-t1)
  Out1 : Outport
  wires:
  Fcn/1 -> Out1/1
  In1/1 -> Fcn/1

== system GunnerusDP_v1/Environment and Vessel Dynamics/Wave definiton (from MCSim)/wave height and wave frequency/Hs and omega16/omega_p/If Action Subsystem3 ==
  In1 : Inport
  Action Port : ActionPort  ActionType=else
  Out1 : Outport
  wires:
  In1/1 -> Out1/1

== system GunnerusDP_v1/Environment and Vessel Dynamics/Wave definiton (from MCSim)/wave height and wave frequency/Hs and omega17/hs/If Action Subsystem1 ==
  In1 : Inport
  Action Port : ActionPort  ActionType=then
  Out1 : Outport
  wires:
  In1/1 -> Out1/1

== system GunnerusDP_v1/Environment and Vessel Dynamics/Wave definiton (from MCSim)/wave height and wave frequency/Hs and omega17/hs/If Action Subsystem2 ==
  In1 : Inport
  Action Port : ActionPort  ActionType=elseif
  Fcn : Fcn  Expr=v1-(v1-v2)/(t2-t1)*(u[1]-t1)
  Out1 : Outport
  wires:
  Fcn/1 -> Out1/1
  In1/1 -> Fcn/1

== system GunnerusDP_v1/Environment and Vessel Dynamics/Wave definiton (from MCSim)/wave height and wave frequency/Hs and omega17/hs/If Action Subsystem3 ==
  In1 : Inport
  Action Port : ActionPort  ActionType=else
  Out1 : Outport
  wires:
  In1/1 -> Out1/1

== system GunnerusDP_v1/Environment and Vessel Dynamics/Wave definiton (from MCSim)/wave height and wave frequency/Hs and omega17/omega_p/If Action Subsystem1 ==
  In1 : Inport
  Action Port : ActionPort  ActionType=then
  Out1 : Outport
  wires:
  In1/1 -> Out1/1

== system GunnerusDP_v1/Environment and Vessel Dynamics/Wave definiton (from MCSim)/wave height and wave frequency/Hs and omega17/omega_p/If Action Subsystem2 ==
  In1 : Inport
  Action Port : ActionPort  ActionType=elseif
  Fcn : Fcn  Expr=v1-(v1-v2)/(t2-t1)*(u[1]-t1)
  Out1 : Outport
  wires:
  In1/1 -> Fcn/1
  Fcn/1 -> Out1/1

== system GunnerusDP_v1/Environment and Vessel Dynamics/Wave definiton (from MCSim)/wave height and wave frequency/Hs and omega17/omega_p/If Action Subsystem3 ==
  In1 : Inport
  Action Port : ActionPort  ActionType=else
  Out1 : Outport
  wires:
  In1/1 -> Out1/1

== system GunnerusDP_v1/Environment and Vessel Dynamics/Wave definiton (from MCSim)/wave height and wave frequency/Hs and omega18/hs/If Action Subsystem1 ==
  In1 : Inport
  Action Port : ActionPort  ActionType=then
  Out1 : Outport
  wires:
  In1/1 -> Out1/1

== system GunnerusDP_v1/Environment and Vessel Dynamics/Wave definiton (from MCSim)/wave height and wave frequency/Hs and omega18/hs/If Action Subsystem2 ==
  In1 : Inport
  Action Port : ActionPort  ActionType=elseif
  Fcn : Fcn  Expr=v1-(v1-v2)/(t2-t1)*(u[1]-t1)
  Out1 : Outport
  wires:
  In1/1 -> Fcn/1
  Fcn/1 -> Out1/1

== system GunnerusDP_v1/Environment and Vessel Dynamics/Wave definiton (from MCSim)/wave height and wave frequency/Hs and omega18/hs/If Action Subsystem3 ==
  In1 : Inport
  Action Port : ActionPort  ActionType=else
  Out1 : Outport
  wires:
  In1/1 -> Out1/1

== system GunnerusDP_v1/Environment and Vessel Dynamics/Wave definiton (from MCSim)/wave height and wave frequency/Hs and omega18/omega_p/If Action Subsystem1 ==
  In1 : Inport
  Action Port : ActionPort  ActionType=then
  Out1 : Outport
  wires:
  In1/1 -> Out1/1

== system GunnerusDP_v1/Environment and Vessel Dynamics/Wave definiton (from MCSim)/wave height and wave frequency/Hs and omega18/omega_p/If Action Subsystem2 ==
  In1 : Inport
  Action Port : ActionPort  ActionType=elseif
  Fcn : Fcn  Expr=v1-(v1-v2)/(t2-t1)*(u[1]-t1)
  Out1 : Outport
  wires:
  Fcn/1 -> Out1/1
  In1/1 -> Fcn/1

== system GunnerusDP_v1/Environment and Vessel Dynamics/Wave definiton (from MCSim)/wave height and wave frequency/Hs and omega18/omega_p/If Action Subsystem3 ==
  In1 : Inport
  Action Port : ActionPort  ActionType=else
  Out1 : Outport
  wires:
  In1/1 -> Out1/1

== system GunnerusDP_v1/Environment and Vessel Dynamics/Wave definiton (from MCSim)/wave height and wave frequency/Hs and omega19/hs/If Action Subsystem1 ==
  In1 : Inport
  Action Port : ActionPort  ActionType=then
  Out1 : Outport
  wires:
  In1/1 -> Out1/1

== system GunnerusDP_v1/Environment and Vessel Dynamics/Wave definiton (from MCSim)/wave height and wave frequency/Hs and omega19/hs/If Action Subsystem2 ==
  In1 : Inport
  Action Port : ActionPort  ActionType=elseif
  Fcn : Fcn  Expr=v1-(v1-v2)/(t2-t1)*(u[1]-t1)
  Out1 : Outport
  wires:
  Fcn/1 -> Out1/1
  In1/1 -> Fcn/1

== system GunnerusDP_v1/Environment and Vessel Dynamics/Wave definiton (from MCSim)/wave height and wave frequency/Hs and omega19/hs/If Action Subsystem3 ==
  In1 : Inport
  Action Port : ActionPort  ActionType=else
  Out1 : Outport
  wires:
  In1/1 -> Out1/1

== system GunnerusDP_v1/Environment and Vessel Dynamics/Wave definiton (from MCSim)/wave height and wave frequency/Hs and omega19/omega_p/If Action Subsystem1 ==
  In1 : Inport
  Action Port : ActionPort  ActionType=then
  Out1 : Outport
  wires:
  In1/1 -> Out1/1

== system GunnerusDP_v1/Environment and Vessel Dynamics/Wave definiton (from MCSim)/wave height and wave frequency/Hs and omega19/omega_p/If Action Subsystem2 ==
  In1 : Inport
  Action Port : ActionPort  ActionType=elseif
  Fcn : Fcn  Expr=v1-(v1-v2)/(t2-t1)*(u[1]-t1)
  Out1 : Outport
  wires:
  In1/1 -> Fcn/1
  Fcn/1 -> Out1/1

== system GunnerusDP_v1/Environment and Vessel Dynamics/Wave definiton (from MCSim)/wave height and wave frequency/Hs and omega19/omega_p/If Action Subsystem3 ==
  In1 : Inport
  Action Port : ActionPort  ActionType=else
  Out1 : Outport
  wires:
  In1/1 -> Out1/1

== system GunnerusDP_v1/Environment and Vessel Dynamics/Wave definiton (from MCSim)/wave height and wave frequency/Hs and omega2/hs/If Action Subsystem1 ==
  In1 : Inport
  Action Port : ActionPort  ActionType=then
  Out1 : Outport
  wires:
  In1/1 -> Out1/1

== system GunnerusDP_v1/Environment and Vessel Dynamics/Wave definiton (from MCSim)/wave height and wave frequency/Hs and omega2/hs/If Action Subsystem2 ==
  In1 : Inport
  Action Port : ActionPort  ActionType=elseif
  Fcn : Fcn  Expr=v1-(v1-v2)/(t2-t1)*(u[1]-t1)
  Out1 : Outport
  wires:
  Fcn/1 -> Out1/1
  In1/1 -> Fcn/1

== system GunnerusDP_v1/Environment and Vessel Dynamics/Wave definiton (from MCSim)/wave height and wave frequency/Hs and omega2/hs/If Action Subsystem3 ==
  In1 : Inport
  Action Port : ActionPort  ActionType=else
  Out1 : Outport
  wires:
  In1/1 -> Out1/1

== system GunnerusDP_v1/Environment and Vessel Dynamics/Wave definiton (from MCSim)/wave height and wave frequency/Hs and omega2/omega_p/If Action Subsystem1 ==
  In1 : Inport
  Action Port : ActionPort  ActionType=then
  Out1 : Outport
  wires:
  In1/1 -> Out1/1

== system GunnerusDP_v1/Environment and Vessel Dynamics/Wave definiton (from MCSim)/wave height and wave frequency/Hs and omega2/omega_p/If Action Subsystem2 ==
  In1 : Inport
  Action Port : ActionPort  ActionType=elseif
  Fcn : Fcn  Expr=v1-(v1-v2)/(t2-t1)*(u[1]-t1)
  Out1 : Outport
  wires:
  In1/1 -> Fcn/1
  Fcn/1 -> Out1/1

== system GunnerusDP_v1/Environment and Vessel Dynamics/Wave definiton (from MCSim)/wave height and wave frequency/Hs and omega2/omega_p/If Action Subsystem3 ==
  In1 : Inport
  Action Port : ActionPort  ActionType=else
  Out1 : Outport
  wires:
  In1/1 -> Out1/1

== system GunnerusDP_v1/Environment and Vessel Dynamics/Wave definiton (from MCSim)/wave height and wave frequency/Hs and omega20/hs/If Action Subsystem1 ==
  In1 : Inport
  Action Port : ActionPort  ActionType=then
  Out1 : Outport
  wires:
  In1/1 -> Out1/1

== system GunnerusDP_v1/Environment and Vessel Dynamics/Wave definiton (from MCSim)/wave height and wave frequency/Hs and omega20/hs/If Action Subsystem2 ==
  In1 : Inport
  Action Port : ActionPort  ActionType=elseif
  Fcn : Fcn  Expr=v1-(v1-v2)/(t2-t1)*(u[1]-t1)
  Out1 : Outport
  wires:
  In1/1 -> Fcn/1
  Fcn/1 -> Out1/1

== system GunnerusDP_v1/Environment and Vessel Dynamics/Wave definiton (from MCSim)/wave height and wave frequency/Hs and omega20/hs/If Action Subsystem3 ==
  In1 : Inport
  Action Port : ActionPort  ActionType=else
  Out1 : Outport
  wires:
  In1/1 -> Out1/1

== system GunnerusDP_v1/Environment and Vessel Dynamics/Wave definiton (from MCSim)/wave height and wave frequency/Hs and omega20/omega_p/If Action Subsystem1 ==
  In1 : Inport
  Action Port : ActionPort  ActionType=then
  Out1 : Outport
  wires:
  In1/1 -> Out1/1

== system GunnerusDP_v1/Environment and Vessel Dynamics/Wave definiton (from MCSim)/wave height and wave frequency/Hs and omega20/omega_p/If Action Subsystem2 ==
  In1 : Inport
  Action Port : ActionPort  ActionType=elseif
  Fcn : Fcn  Expr=v1-(v1-v2)/(t2-t1)*(u[1]-t1)
  Out1 : Outport
  wires:
  Fcn/1 -> Out1/1
  In1/1 -> Fcn/1

== system GunnerusDP_v1/Environment and Vessel Dynamics/Wave definiton (from MCSim)/wave height and wave frequency/Hs and omega20/omega_p/If Action Subsystem3 ==
  In1 : Inport
  Action Port : ActionPort  ActionType=else
  Out1 : Outport
  wires:
  In1/1 -> Out1/1

== system GunnerusDP_v1/Environment and Vessel Dynamics/Wave definiton (from MCSim)/wave height and wave frequency/Hs and omega21/hs/If Action Subsystem1 ==
  In1 : Inport
  Action Port : ActionPort  ActionType=then
  Out1 : Outport
  wires:
  In1/1 -> Out1/1

== system GunnerusDP_v1/Environment and Vessel Dynamics/Wave definiton (from MCSim)/wave height and wave frequency/Hs and omega21/hs/If Action Subsystem2 ==
  In1 : Inport
  Action Port : ActionPort  ActionType=elseif
  Fcn : Fcn  Expr=v1-(v1-v2)/(t2-t1)*(u[1]-t1)
  Out1 : Outport
  wires:
  Fcn/1 -> Out1/1
  In1/1 -> Fcn/1

== system GunnerusDP_v1/Environment and Vessel Dynamics/Wave definiton (from MCSim)/wave height and wave frequency/Hs and omega21/hs/If Action Subsystem3 ==
  In1 : Inport
  Action Port : ActionPort  ActionType=else
  Out1 : Outport
  wires:
  In1/1 -> Out1/1

== system GunnerusDP_v1/Environment and Vessel Dynamics/Wave definiton (from MCSim)/wave height and wave frequency/Hs and omega21/omega_p/If Action Subsystem1 ==
  In1 : Inport
  Action Port : ActionPort  ActionType=then
  Out1 : Outport
  wires:
  In1/1 -> Out1/1

== system GunnerusDP_v1/Environment and Vessel Dynamics/Wave definiton (from MCSim)/wave height and wave frequency/Hs and omega21/omega_p/If Action Subsystem2 ==
  In1 : Inport
  Action Port : ActionPort  ActionType=elseif
  Fcn : Fcn  Expr=v1-(v1-v2)/(t2-t1)*(u[1]-t1)
  Out1 : Outport
  wires:
  In1/1 -> Fcn/1
  Fcn/1 -> Out1/1

== system GunnerusDP_v1/Environment and Vessel Dynamics/Wave definiton (from MCSim)/wave height and wave frequency/Hs and omega21/omega_p/If Action Subsystem3 ==
  In1 : Inport
  Action Port : ActionPort  ActionType=else
  Out1 : Outport
  wires:
  In1/1 -> Out1/1

== system GunnerusDP_v1/Environment and Vessel Dynamics/Wave definiton (from MCSim)/wave height and wave frequency/Hs and omega22/hs/If Action Subsystem1 ==
  In1 : Inport
  Action Port : ActionPort  ActionType=then
  Out1 : Outport
  wires:
  In1/1 -> Out1/1

== system GunnerusDP_v1/Environment and Vessel Dynamics/Wave definiton (from MCSim)/wave height and wave frequency/Hs and omega22/hs/If Action Subsystem2 ==
  In1 : Inport
  Action Port : ActionPort  ActionType=elseif
  Fcn : Fcn  Expr=v1-(v1-v2)/(t2-t1)*(u[1]-t1)
  Out1 : Outport
  wires:
  In1/1 -> Fcn/1
  Fcn/1 -> Out1/1

== system GunnerusDP_v1/Environment and Vessel Dynamics/Wave definiton (from MCSim)/wave height and wave frequency/Hs and omega22/hs/If Action Subsystem3 ==
  In1 : Inport
  Action Port : ActionPort  ActionType=else
  Out1 : Outport
  wires:
  In1/1 -> Out1/1

== system GunnerusDP_v1/Environment and Vessel Dynamics/Wave definiton (from MCSim)/wave height and wave frequency/Hs and omega22/omega_p/If Action Subsystem1 ==
  In1 : Inport
  Action Port : ActionPort  ActionType=then
  Out1 : Outport
  wires:
  In1/1 -> Out1/1

== system GunnerusDP_v1/Environment and Vessel Dynamics/Wave definiton (from MCSim)/wave height and wave frequency/Hs and omega22/omega_p/If Action Subsystem2 ==
  In1 : Inport
  Action Port : ActionPort  ActionType=elseif
  Fcn : Fcn  Expr=v1-(v1-v2)/(t2-t1)*(u[1]-t1)
  Out1 : Outport
  wires:
  Fcn/1 -> Out1/1
  In1/1 -> Fcn/1

== system GunnerusDP_v1/Environment and Vessel Dynamics/Wave definiton (from MCSim)/wave height and wave frequency/Hs and omega22/omega_p/If Action Subsystem3 ==
  In1 : Inport
  Action Port : ActionPort  ActionType=else
  Out1 : Outport
  wires:
  In1/1 -> Out1/1

== system GunnerusDP_v1/Environment and Vessel Dynamics/Wave definiton (from MCSim)/wave height and wave frequency/Hs and omega23/hs/If Action Subsystem1 ==
  In1 : Inport
  Action Port : ActionPort  ActionType=then
  Out1 : Outport
  wires:
  In1/1 -> Out1/1

== system GunnerusDP_v1/Environment and Vessel Dynamics/Wave definiton (from MCSim)/wave height and wave frequency/Hs and omega23/hs/If Action Subsystem2 ==
  In1 : Inport
  Action Port : ActionPort  ActionType=elseif
  Fcn : Fcn  Expr=v1-(v1-v2)/(t2-t1)*(u[1]-t1)
  Out1 : Outport
  wires:
  Fcn/1 -> Out1/1
  In1/1 -> Fcn/1

== system GunnerusDP_v1/Environment and Vessel Dynamics/Wave definiton (from MCSim)/wave height and wave frequency/Hs and omega23/hs/If Action Subsystem3 ==
  In1 : Inport
  Action Port : ActionPort  ActionType=else
  Out1 : Outport
  wires:
  In1/1 -> Out1/1

== system GunnerusDP_v1/Environment and Vessel Dynamics/Wave definiton (from MCSim)/wave height and wave frequency/Hs and omega23/omega_p/If Action Subsystem1 ==
  In1 : Inport
  Action Port : ActionPort  ActionType=then
  Out1 : Outport
  wires:
  In1/1 -> Out1/1

== system GunnerusDP_v1/Environment and Vessel Dynamics/Wave definiton (from MCSim)/wave height and wave frequency/Hs and omega23/omega_p/If Action Subsystem2 ==
  In1 : Inport
  Action Port : ActionPort  ActionType=elseif
  Fcn : Fcn  Expr=v1-(v1-v2)/(t2-t1)*(u[1]-t1)
  Out1 : Outport
  wires:
  In1/1 -> Fcn/1
  Fcn/1 -> Out1/1

== system GunnerusDP_v1/Environment and Vessel Dynamics/Wave definiton (from MCSim)/wave height and wave frequency/Hs and omega23/omega_p/If Action Subsystem3 ==
  In1 : Inport
  Action Port : ActionPort  ActionType=else
  Out1 : Outport
  wires:
  In1/1 -> Out1/1
